simulink library "MK_K"  (R2025a)
settings: Solver=VariableStepAuto  StartTime=0.0  StopTime=10.0  RelTol=1e-3
settings Model: Creator=Szalay  LastModifiedBy=Szalay

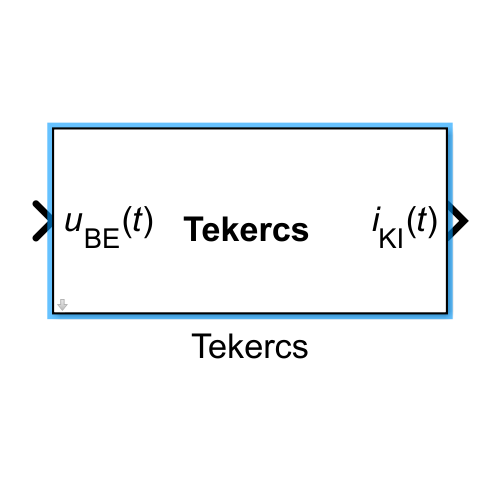
[thumbnail: Simulink's stored preview of the top-level diagram]
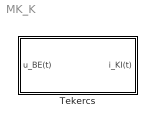
== system MK_K ==
  Tekercs : Subsystem  mask(Tekercs){L=1e-3, R=1, i_0=0.5}
      mask prompts: L "Öninduktivitás (H)"; R "Ellenállás (Ohm)"; i_0 "Kezdeti áramerősség (A)"
      mask help: Lineáris mágnesezettségű tekercs modell (RL-tag).
      mask DialogControl ParameterGroupVar Prompt: Modellparaméterek
      mask DialogControl Container3 Prompt: Kezdeti érték
      mask Display:
      | % Felirat
      | text( ...
      |     0.5, 0.5, '{\bfTekercs}', ...
      |     'HorizontalAlignment', 'center', ...
      |     'Interpreter', 'tex' ...
      |     );
      | 
      | % Csatlakozók
      | port_label( ...
      |     'input', 1, '{\itu}_{BE}({\itt})', ...
      |     'texmode', 'on' ...
      |     );
      | port_label( ...
      |     'output', 1, '{\iti}_{KI}({\itt})', ...
      |     'texmode', 'on' ...
      |     );

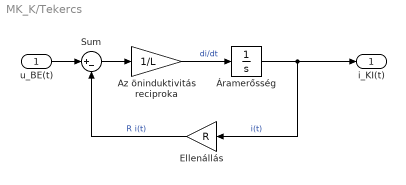
== system MK_K/Tekercs ==
  u_BE(t) : Inport
  Az öninduktivitás reciproka : Gain  Gain=1/L
  Ellenállás : Gain  Gain=R
  Sum : Sum  Inputs=|+-
  Áramerősség : Integrator  InitialCondition=i_0
  i_KI(t) : Outport
  wires:
  Áramerősség/1 -> i_KI(t)/1, Ellenállás/1  "i(t)"
  Az öninduktivitás reciproka/1 -> Áramerősség/1  "di/dt"
  Ellenállás/1 -> Sum/2  "R i(t)"
  Sum/1 -> Az öninduktivitás reciproka/1
  u_BE(t)/1 -> Sum/1
